simulink model "Joint_State_Space_Simulation"  (R2019a)
settings: Solver=VariableStepAuto  StartTime=0.0  StopTime=10  RelTol=1e-3
values from neighbouring files (symbols this model uses):
  A = 1/5    (= 0.2)    [Joint_Init.m]    (also in Joint_State_Space.m = [0, 1, 0, 0)
  B = 0*Alpha    [Joint_SI.m]    (also in Joint_SI_noArm.m = 0*R; Joint_State_Space.m = [0, f, 0, -f])
  C = [1, 0, 0, 0 ... (first row only)    [Joint_State_Space.m]
  G = 0*dTheta_tf    [Joint_SI_Dtheta.m]    (also in Joint_State_Space.m = [1, 0, 0, 0])
  K = mean(B_log(2:4))    [Joint_SI.m]    (also in Joint_SI_Dtheta.m = mean(G_log(3:15)); Joint_SI_noArm.m = mean(B_log(2:5)); Joint_State_Space.m = K_joint(1:2))
  Ki = -K_joint(3)    [Joint_State_Space.m]
settings Model: Creator=QuarcUser  LastModifiedBy=QuarcUser

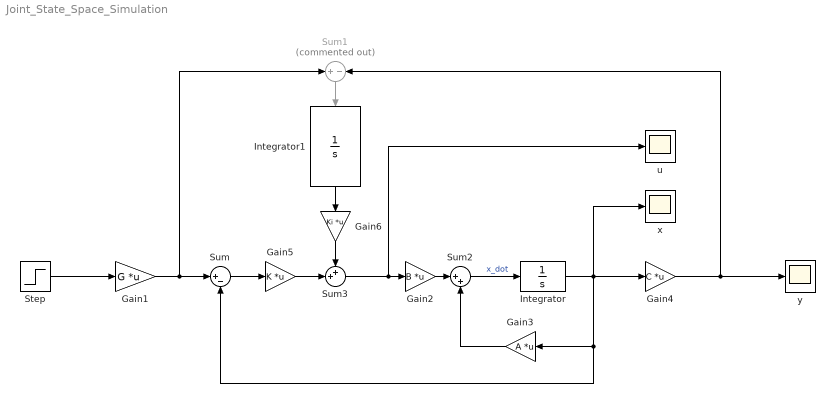
== system Joint_State_Space_Simulation ==
  Gain1 : Gain  Gain=G  Multiplication=Matrix(K*u)
  Gain2 : Gain  Gain=B  Multiplication=Matrix(K*u)
  Gain3 : Gain  Gain=A  Multiplication=Matrix(K*u)
  Gain4 : Gain  Gain=C  Multiplication=Matrix(K*u)
  Gain5 : Gain  Gain=K  Multiplication=Matrix(K*u)
  Gain6 : Gain  Gain=Ki  Multiplication=Matrix(K*u)
  Integrator : Integrator  InitialCondition=[0;0]
  Integrator1 : Integrator  InitialCondition=[0;0]
  Step : Step  SampleTime=.002
  Sum : Sum  Inputs=|+-
  Sum1 : Sum  Commented=on  Inputs=+-
  Sum2 : Sum  Inputs=|++
  Sum3 : Sum  Inputs=++|
  u : Scope
  x : Scope
  y : Scope
  wires:
  Sum/1 -> Gain5/1
  Gain2/1 -> Sum2/1
  Sum2/1 -> Integrator/1  "x_dot"
  Gain3/1 -> Sum2/2
  Sum1/1 -> Integrator1/1
  Gain4/1 -> y/1, Sum1/2
  Integrator1/1 -> Gain6/1
  Integrator/1 -> Sum/2, Gain3/1, x/1, Gain4/1
  Gain1/1 -> Sum1/1, Sum/1
  Step/1 -> Gain1/1
  Sum3/1 -> u/1, Gain2/1
  Gain5/1 -> Sum3/2
  Gain6/1 -> Sum3/1
